simulink model "l5"  (R2012b)
settings: Solver=ode45  StartTime=0.0  StopTime=480  RelTol=1e-3
undefined symbols (not defined in the file): des, gcbh
settings Model: Creator=Student  LastModifiedBy=gick

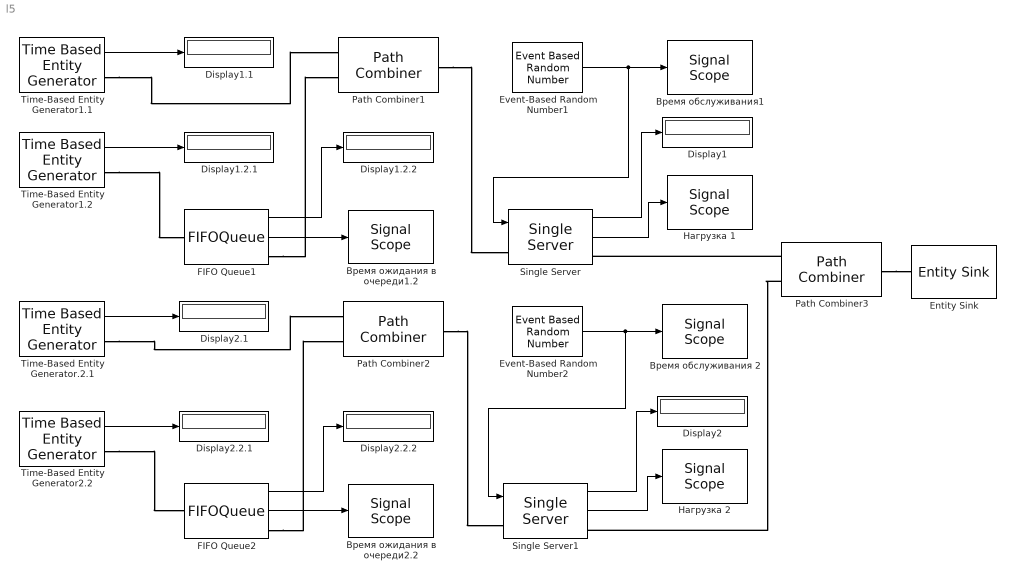
== system l5 ==
  Display1 : Display
  Display1.1 : Display
  Display1.2.1 : Display
  Display1.2.2 : Display
  Display2 : Display
  Display2.1 : Display
  Display2.2.1 : Display
  Display2.2.2 : Display
  Entity Sink : EntitySink
  Event-Based Random Number1 : EventBasedRandomNumber  Distribution=Uniform  meanExp=2.5  minUnif=8  maxUnif=14  Seed=12
  Event-Based Random Number2 : EventBasedRandomNumber  Distribution=Uniform  meanExp=3  minUnif=6  maxUnif=7  Seed=12
  FIFO Queue1 : FIFOQueue  Capacity=30  StatNumberDeparted=on  StatAverageWait=on
      settings: OutputPortMap=o0,o2
  FIFO Queue2 : FIFOQueue  Capacity=30  StatNumberDeparted=on  StatAverageWait=on
      settings: OutputPortMap=o0,o2
  Path Combiner1 : PathCombiner  NumberInputPorts=2
  Path Combiner2 : PathCombiner  NumberInputPorts=2
  Path Combiner3 : PathCombiner  NumberInputPorts=2  InputPortPrecedence=Round robin
  Single Server : SingleServer  ServiceTimeFrom=Signal port t  PriorityServiceCompletion=50  StatNumberDeparted=on  StatUtilization=on
      settings: OutputPortMap=o0,o5
  Single Server1 : SingleServer  ServiceTimeFrom=Signal port t  PriorityServiceCompletion=50  StatNumberDeparted=on  StatUtilization=on
      settings: OutputPortMap=o0,o5
  Time-Based Entity Generator.2.1 : TimeBasedEntityGenerator  Distribution=Exponential  Period=20  InitialSeed=12  Mean=25  StatNumberDeparted=on
  Time-Based Entity Generator1.1 : TimeBasedEntityGenerator  Distribution=Exponential  Period=20  InitialSeed=12  Mean=50  StatNumberDeparted=on
  Time-Based Entity Generator1.2 : TimeBasedEntityGenerator  Distribution=Exponential  Period=3  InitialSeed=12  Mean=30  StatNumberDeparted=on
  Time-Based Entity Generator2.2 : TimeBasedEntityGenerator  Distribution=Exponential  Period=3  InitialSeed=12  Mean=15  PriorityEntityGeneration=500  StatNumberDeparted=on
  Время обслуживания 2 : SignalScope  LoadFcn=des.scope.CallbackSupport('seLoadFcn',gcbh)  StartFcn=des.scope.CallbackSupport('seStartFcn',gcbh)  StopFcn=des.scope.CallbackSupport('seStopFcn',gcbh)  ShowCountPlotted=on
      settings: CopyFcn=des.scope.CallbackSupport('seCopyFcn',gcbh)  DeleteFcn=des.scope.CallbackSupport('seDeleteFcn',gcbh)  PreSaveFcn=des.scope.CallbackSupport('sePreSaveFcn',gcbh)  NameChangeFcn=des.scope.CallbackSupport('seNameChangeFcn',gcbh)  OpenFcn=des.scope.CallbackSupport('seOpenFcn',gcbh)
  Время обслуживания1 : SignalScope  LoadFcn=des.scope.CallbackSupport('seLoadFcn',gcbh)  StartFcn=des.scope.CallbackSupport('seStartFcn',gcbh)  StopFcn=des.scope.CallbackSupport('seStopFcn',gcbh)  ShowCountPlotted=on
      settings: CopyFcn=des.scope.CallbackSupport('seCopyFcn',gcbh)  DeleteFcn=des.scope.CallbackSupport('seDeleteFcn',gcbh)  PreSaveFcn=des.scope.CallbackSupport('sePreSaveFcn',gcbh)  NameChangeFcn=des.scope.CallbackSupport('seNameChangeFcn',gcbh)  OpenFcn=des.scope.CallbackSupport('seOpenFcn',gcbh)
  Время ожидания в очереди1.2 : SignalScope  LoadFcn=des.scope.CallbackSupport('seLoadFcn',gcbh)  StartFcn=des.scope.CallbackSupport('seStartFcn',gcbh)  StopFcn=des.scope.CallbackSupport('seStopFcn',gcbh)  ShowCountPlotted=on
      settings: CopyFcn=des.scope.CallbackSupport('seCopyFcn',gcbh)  DeleteFcn=des.scope.CallbackSupport('seDeleteFcn',gcbh)  PreSaveFcn=des.scope.CallbackSupport('sePreSaveFcn',gcbh)  NameChangeFcn=des.scope.CallbackSupport('seNameChangeFcn',gcbh)  OpenFcn=des.scope.CallbackSupport('seOpenFcn',gcbh)
  Время ожидания в очереди2.2 : SignalScope  LoadFcn=des.scope.CallbackSupport('seLoadFcn',gcbh)  StartFcn=des.scope.CallbackSupport('seStartFcn',gcbh)  StopFcn=des.scope.CallbackSupport('seStopFcn',gcbh)  ShowCountPlotted=on
      settings: CopyFcn=des.scope.CallbackSupport('seCopyFcn',gcbh)  DeleteFcn=des.scope.CallbackSupport('seDeleteFcn',gcbh)  PreSaveFcn=des.scope.CallbackSupport('sePreSaveFcn',gcbh)  NameChangeFcn=des.scope.CallbackSupport('seNameChangeFcn',gcbh)  OpenFcn=des.scope.CallbackSupport('seOpenFcn',gcbh)
  Нагрузка 1 : SignalScope  LoadFcn=des.scope.CallbackSupport('seLoadFcn',gcbh)  StartFcn=des.scope.CallbackSupport('seStartFcn',gcbh)  StopFcn=des.scope.CallbackSupport('seStopFcn',gcbh)  XMax=640  ShowCountPlotted=on
      settings: CopyFcn=des.scope.CallbackSupport('seCopyFcn',gcbh)  DeleteFcn=des.scope.CallbackSupport('seDeleteFcn',gcbh)  PreSaveFcn=des.scope.CallbackSupport('sePreSaveFcn',gcbh)  NameChangeFcn=des.scope.CallbackSupport('seNameChangeFcn',gcbh)  OpenFcn=des.scope.CallbackSupport('seOpenFcn',gcbh)
  Нагрузка 2 : SignalScope  LoadFcn=des.scope.CallbackSupport('seLoadFcn',gcbh)  StartFcn=des.scope.CallbackSupport('seStartFcn',gcbh)  StopFcn=des.scope.CallbackSupport('seStopFcn',gcbh)  ShowCountPlotted=on
      settings: CopyFcn=des.scope.CallbackSupport('seCopyFcn',gcbh)  DeleteFcn=des.scope.CallbackSupport('seDeleteFcn',gcbh)  PreSaveFcn=des.scope.CallbackSupport('sePreSaveFcn',gcbh)  NameChangeFcn=des.scope.CallbackSupport('seNameChangeFcn',gcbh)  OpenFcn=des.scope.CallbackSupport('seOpenFcn',gcbh)
  wires:
  Time-Based Entity Generator1.2/1 -> Display1.2.1/1
  Time-Based Entity Generator1.1/1 -> Display1.1/1
  FIFO Queue1/1 -> Display1.2.2/1
  FIFO Queue1/2 -> Время ожидания в очереди1.2/1
  Event-Based Random Number1/1 -> Время обслуживания1/1, Single Server/1
  Single Server/1 -> Display1/1
  Single Server/2 -> Нагрузка 1/1
  Time-Based Entity Generator2.2/1 -> Display2.2.1/1
  FIFO Queue2/1 -> Display2.2.2/1
  Time-Based Entity Generator.2.1/1 -> Display2.1/1
  FIFO Queue2/2 -> Время ожидания в очереди2.2/1
  Event-Based Random Number2/1 -> Время обслуживания 2/1, Single Server1/1
  Single Server1/1 -> Display2/1
  Single Server1/2 -> Нагрузка 2/1
  connections:
  Time-Based Entity Generator1.2/RConn1 -- FIFO Queue1/LConn1
  FIFO Queue1/RConn1 -- Path Combiner1/LConn2
  Time-Based Entity Generator1.1/RConn1 -- Path Combiner1/LConn1
  Path Combiner1/RConn1 -- Single Server/LConn1
  Path Combiner3/LConn1 -- Single Server/RConn1
  Path Combiner3/RConn1 -- Entity Sink/LConn1
  Time-Based Entity Generator2.2/RConn1 -- FIFO Queue2/LConn1
  FIFO Queue2/RConn1 -- Path Combiner2/LConn2
  Time-Based Entity Generator.2.1/RConn1 -- Path Combiner2/LConn1
  Path Combiner2/RConn1 -- Single Server1/LConn1
  Path Combiner3/LConn2 -- Single Server1/RConn1
